simulink model "Schema_Fonctionnel_angle"  (R2025b)
settings: Solver=VariableStepAuto  StartTime=0.0  StopTime=10.0  RelTol=1e-3
values from neighbouring files (symbols this model uses):
  Kdo = 13.4    [script_devoir2.m]
  Kio = 0.6    [script_devoir2.m]
undefined symbols (not defined in the file or in its folder): Kpo
settings Model: Creator=Louis  LastModifiedBy=Louis

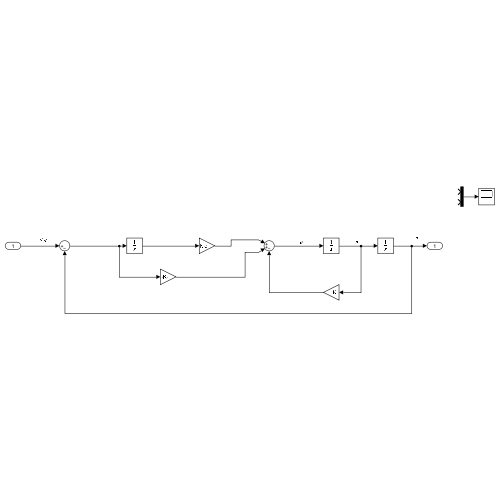
[thumbnail: Simulink's stored preview of the top-level diagram]
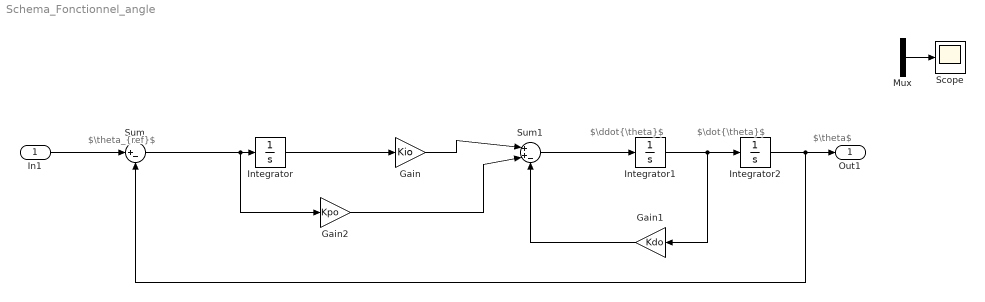
== system Schema_Fonctionnel_angle ==
  note: $\ddot{\theta}$
  note: $\theta$
  note: $\theta_{ref}$
  note: $\dot{\theta}$
  In1 : Inport
  Gain : Gain  Gain=Kio
  Gain1 : Gain  Gain=Kdo
  Gain2 : Gain  Gain=Kpo
  Integrator : Integrator
  Integrator1 : Integrator
  Integrator2 : Integrator
  Mux : Mux  Inputs=2
  Scope : Scope
      settings: ActiveDisplayYMinimum=-1  ActiveDisplayYMaximum=1  DataLoggingVariableName=Y1  DataLoggingSaveFormat=Array
  Sum : Sum  Inputs=|+-
  Sum1 : Sum  Inputs=|++-
  Out1 : Outport
  wires:
  Integrator/1 -> Gain/1
  Gain2/1 -> Sum1/2
  Mux/1 -> Scope/1
  Sum1/1 -> Integrator1/1
  Integrator2/1 -> Out1/1, Sum/2
  Sum/1 -> Gain2/1, Integrator/1
  Gain1/1 -> Sum1/3
  In1/1 -> Sum/1
  Gain/1 -> Sum1/1
  Integrator1/1 -> Gain1/1, Integrator2/1
